simulink model "robot_delta_din_model_lagrange_teorico_prueba"  (R2018b)
settings: Solver=ode3  StartTime=0.0  StopTime=16.625  FixedStep=0.005  RelTol=1e-3  EnableMultiTasking=on
values from neighbouring files (symbols this model uses):
  theta = [-0.0693180218986 0.00226424410725 -4.83793342673e-06 0.00608650555065 -0.253389972154 -1.12828320096 -0.000817462918057 0.000589548664253 0.00594878456256 -1.00496882122 -0.000840049540021 -0.000607800169067 ... (14 elements, 14x1)]    [constantes_ident_lagrange_val_delta_2.mat]
settings Model: Creator=Jairo  LastModifiedBy=jairo
settings DataIOCC: LimitDataPoints=on  SaveFormat=Array
settings OptimizationCC: LifeSpan=inf
settings DebuggingCC: UnderspecifiedInitializationDetection=Classic  MergeDetectMultiDrivingBlocksExec=none  SolverPrmCheckMsg=warning  StateNameClashWarn=warning  SFUnexpectedBacktrackingDiag=warning  SFNoUnconditionalDefaultTransitionDiag=warning  SFExecutionAtInitializationDiag=none
settings HardwareCC: ProdBitPerPointer=32  ProdBitPerSizeT=32  ProdBitPerPtrDiffT=32  ProdLargestAtomicFloat=None  ProdIntDivRoundTo=Undefined  ProdEndianess=Unspecified  ProdWordSize=32  ProdHWDeviceType=32-bit Generic
settings ModelReferenceCC: PropagateSignalLabelsOutOfModel=off
settings SFSimCC: SimUseLocalCustomCode=off
settings RTWCC: RTWUseLocalCustomCode=off
settings CodeAppCC: StateflowObjectComments=on
settings GRTTargetCC: TargetLangStandard=C89/C90 (ANSI)  GeneratePreprocessorConditionals=Disable all
settings ConfigComp: CovMetricSettings=dw  CovHtmlReporting=on  CovSaveCumulativeToWorkspaceVar=on  CovSaveSingleToWorkspaceVar=on  CovExternalEMLEnable=off

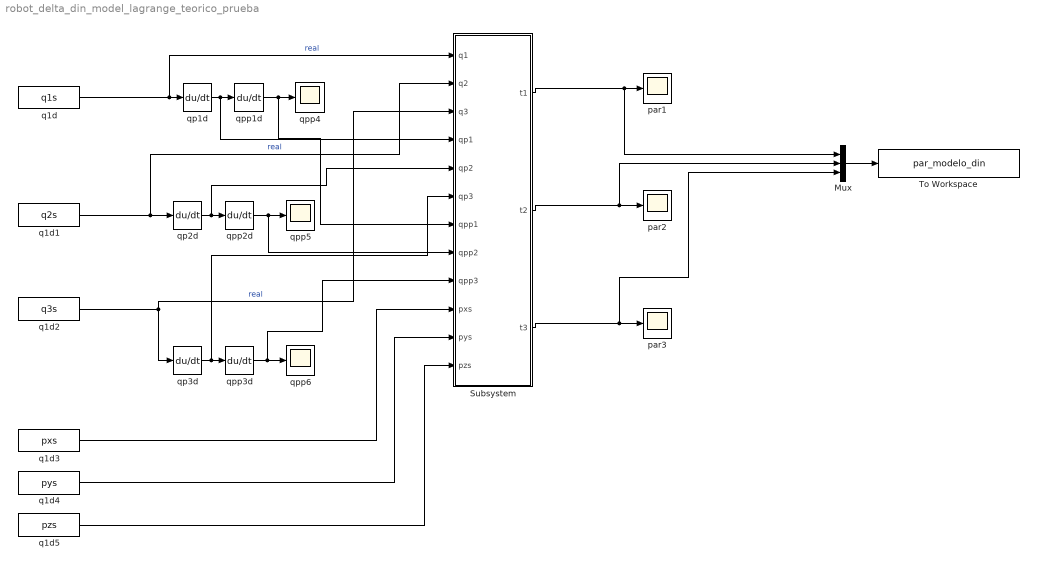
== system robot_delta_din_model_lagrange_teorico_prueba ==
  Mux : Mux  Inputs=3
  Subsystem : Subsystem
  To Workspace : ToWorkspace  VariableName=par_modelo_din  SampleTime=-1
  par1 : Scope
  par2 : Scope
  par3 : Scope
  q1d : FromWorkspace  VariableName=q1s  SampleTime=0.005
  q1d1 : FromWorkspace  VariableName=q2s  SampleTime=0.005
  q1d2 : FromWorkspace  VariableName=q3s  SampleTime=0.005
  q1d3 : FromWorkspace  VariableName=pxs  SampleTime=0.005
  q1d4 : FromWorkspace  VariableName=pys  SampleTime=0.005
  q1d5 : FromWorkspace  VariableName=pzs  SampleTime=0.005
  qp1d : Derivative
  qp2d : Derivative
  qp3d : Derivative
  qpp1d : Derivative
  qpp2d : Derivative
  qpp3d : Derivative
  qpp4 : Scope
  qpp5 : Scope
  qpp6 : Scope
  wires:
  q1d1/1 -> Subsystem/2(q2), qp2d/1  "real"
  qp2d/1 -> Subsystem/5(qp2), qpp2d/1
  qpp2d/1 -> Subsystem/8(qpp2), qpp5/1
  q1d2/1 -> qp3d/1, Subsystem/3(q3)  "real"
  qp3d/1 -> Subsystem/6(qp3), qpp3d/1
  qpp3d/1 -> Subsystem/9(qpp3), qpp6/1
  q1d/1 -> Subsystem/1(q1), qp1d/1  "real"
  qp1d/1 -> Subsystem/4(qp1), qpp1d/1
  qpp1d/1 -> Subsystem/7(qpp1), qpp4/1
  Subsystem/1(t1) -> Mux/1, par1/1
  Subsystem/2(t2) -> Mux/2, par2/1
  Mux/1 -> To Workspace/1
  Subsystem/3(t3) -> Mux/3, par3/1
  q1d3/1 -> Subsystem/10(pxs)
  q1d4/1 -> Subsystem/11(pys)
  q1d5/1 -> Subsystem/12(pzs)

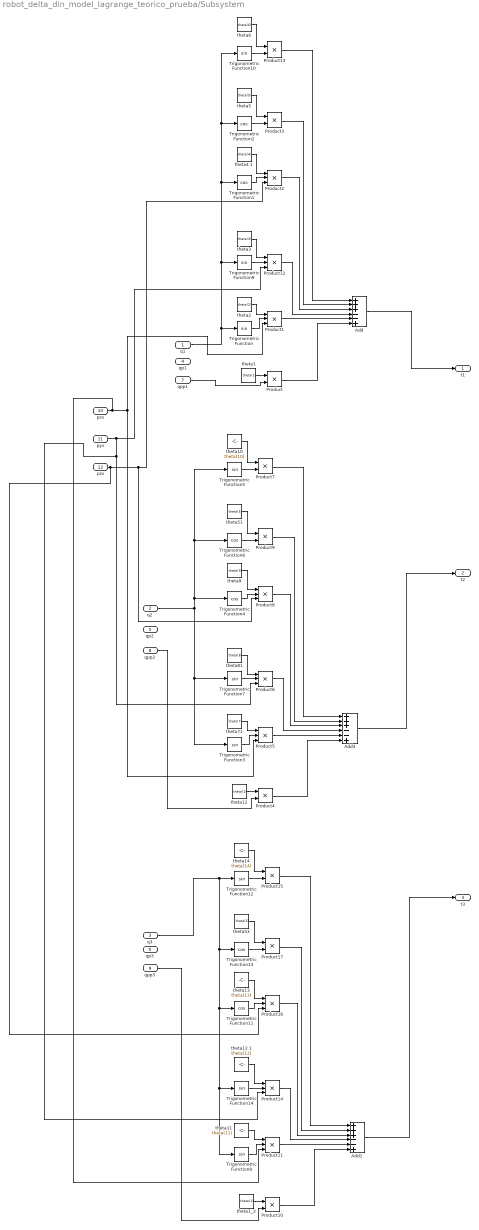
== system robot_delta_din_model_lagrange_teorico_prueba/Subsystem ==
  q1 : Inport
  q2 : Inport  Port=2
  q3 : Inport  Port=3
  qp1 : Inport  Port=4
  qp2 : Inport  Port=5
  qp3 : Inport  Port=6
  qpp1 : Inport  Port=7
  qpp2 : Inport  Port=8
  qpp3 : Inport  Port=9
  pxs : Inport  Port=10
  pys : Inport  Port=11
  pzs : Inport  Port=12
  Add : Sum  Inputs=+++--+
  Add1 : Sum  Inputs=+++--+
  Add3 : Sum  Inputs=+++--+
  Product{,3..4,7,9..10,13,15,17} (9 alike) : Product
  Product{1..2,5..6,8,11..12,14,16} (9 alike) : Product  Inputs=3
  Trigonometric Function{,3,5,7..10,12,14} (9 alike) : Trigonometry
  Trigonometric Function{1..2,4,6,11,13} (6 alike) : Trigonometry  Operator=cos
  theta1 : Constant  Value=theta(1)
  theta10 : Constant  Value=theta(10)
  theta11 : Constant  Value=theta(11)
  theta12 : Constant  Value=theta(1)
  theta12 1 : Constant  Value=theta(12)
  theta13 : Constant  Value=theta(13)
  theta14 : Constant  Value=theta(14)
  theta1_3 : Constant  Value=theta(1)
  theta2 : Constant  Value=theta(2)
  "theta3 " : Constant  Value=theta(3)
  theta4 1 : Constant  Value=theta(4)
  theta5 : Constant  Value=theta(5)
  theta51 : Constant  Value=theta(5)
  theta53 : Constant  Value=theta(5)
  theta6 : Constant  Value=theta(6)
  theta71 : Constant  Value=theta(7)
  theta81 : Constant  Value=theta(8)
  theta9 : Constant  Value=theta(9)
  t1 : Outport
  t2 : Outport  Port=2
  t3 : Outport  Port=3
  wires:
  Trigonometric Function/1 -> Product1/2
  theta2/1 -> Product1/1
  q1/1 -> Trigonometric Function10/1, Trigonometric Function2/1, Trigonometric Function1/1, Trigonometric Function9/1, Trigonometric Function/1
  Add/1 -> t1/1
  theta1/1 -> Product/1
  qpp1/1 -> Product/2
  Product/1 -> Add/6
  Product1/1 -> Add/5
  Trigonometric Function9/1 -> Product12/2
  "theta3 "/1 -> Product12/1
  Product12/1 -> Add/4
  Trigonometric Function1/1 -> Product2/2
  theta4 1/1 -> Product2/1
  Product2/1 -> Add/3
  Trigonometric Function2/1 -> Product3/2
  theta5/1 -> Product3/1
  Product3/1 -> Add/2
  Trigonometric Function10/1 -> Product13/2
  theta6/1 -> Product13/1
  Product13/1 -> Add/1
  Trigonometric Function3/1 -> Product5/2
  theta71/1 -> Product5/1
  q2/1 -> Trigonometric Function3/1, Trigonometric Function7/1, Trigonometric Function5/1, Trigonometric Function6/1, Trigonometric Function4/1
  theta12/1 -> Product4/1
  Product4/1 -> Add3/6
  Product5/1 -> Add3/5
  Trigonometric Function7/1 -> Product6/2
  theta81/1 -> Product6/1
  Product6/1 -> Add3/4
  Trigonometric Function4/1 -> Product8/2
  theta9/1 -> Product8/1
  Product8/1 -> Add3/3
  Trigonometric Function6/1 -> Product9/2
  theta51/1 -> Product9/1
  Product9/1 -> Add3/2
  Trigonometric Function5/1 -> Product7/2
  theta10/1 -> Product7/1
  Product7/1 -> Add3/1
  Add3/1 -> t2/1
  qpp2/1 -> Product4/2
  Trigonometric Function8/1 -> Product11/2
  theta11/1 -> Product11/1
  q3/1 -> Trigonometric Function8/1, Trigonometric Function14/1, Trigonometric Function11/1, Trigonometric Function13/1, Trigonometric Function12/1
  theta1_3/1 -> Product10/1
  qpp3/1 -> Product10/2
  Product10/1 -> Add1/6
  Product11/1 -> Add1/5
  Trigonometric Function14/1 -> Product14/2
  theta12 1/1 -> Product14/1
  Product14/1 -> Add1/4
  Trigonometric Function11/1 -> Product16/2
  theta13/1 -> Product16/1
  Product16/1 -> Add1/3
  Trigonometric Function13/1 -> Product17/2
  theta53/1 -> Product17/1
  Product17/1 -> Add1/2
  Trigonometric Function12/1 -> Product15/2
  theta14/1 -> Product15/1
  Product15/1 -> Add1/1
  Add1/1 -> t3/1
  pxs/1 -> Product11/3, Product1/3, Product5/3
  pys/1 -> Product14/3, Product6/3, Product12/3
  pzs/1 -> Product16/3, Product8/3, Product2/3
